simulink subsystem "Control_Attitude_Thrust"  (R2025b)
settings: Solver=VariableStepAuto  StartTime=0.0  StopTime=10.0  RelTol=1e-3
undefined symbols (not defined in the file): g0, Ktheta, Kthetadot, StabTrimPos, Tdoublet
libraries: simulink_extras x7
settings Model: Creator=invrt  LastModifiedBy=cdriggs

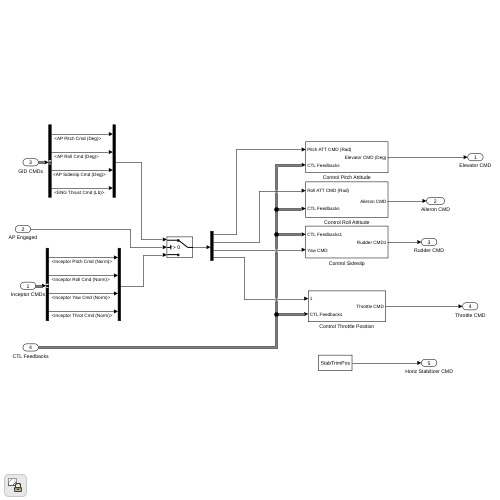
[thumbnail: Simulink's stored preview of the top-level diagram]
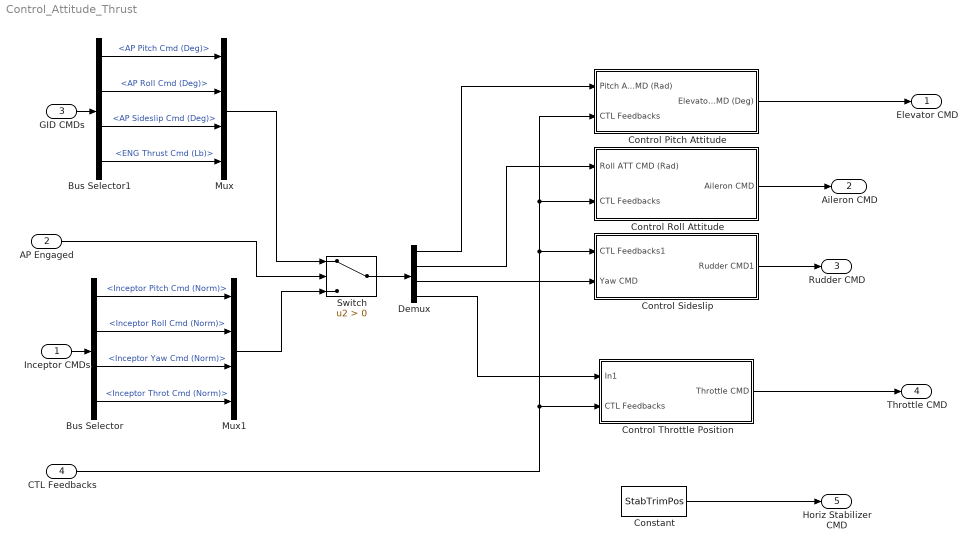
== system Control_Attitude_Thrust ==
  Inceptor CMDs : Inport
  AP Engaged : Inport  Port=2
  GID CMDs : Inport  Port=3
  CTL Feedbacks : Inport  Port=4
  Bus Selector : BusSelector  OutputSignals=Inceptor Pitch Cmd (Norm),Inceptor Roll Cmd (Norm),Inceptor Yaw Cmd (Norm),Inceptor Throt Cmd (Norm)
  Bus Selector1 : BusSelector  OutputSignals=AP Pitch Cmd (Deg),AP Roll Cmd (Deg),AP Sideslip Cmd (Deg),ENG Thrust Cmd (Lb)
  Constant : Constant  Value=StabTrimPos
  Control Pitch Attitude : Subsystem
  Control Roll Attitude : Subsystem
  Control Sideslip : Subsystem
  Control Throttle Position : Subsystem
  Demux : Demux
  Mux : Mux
  Mux1 : Mux
  Switch : Switch  Criteria=u2 > Threshold  SaturateOnIntegerOverflow=off  InputSameDT=off
  Elevator CMD : Outport
  Aileron CMD : Outport  Port=2
  Rudder CMD : Outport  Port=3
  Throttle CMD : Outport  Port=4
  Horiz Stabilizer CMD : Outport  Port=5
  wires:
  Inceptor CMDs/1 -> Bus Selector/1
  Bus Selector/1 -> Mux1/1  "<Inceptor Pitch Cmd (Norm)>"
  GID CMDs/1 -> Bus Selector1/1
  Bus Selector1/4 -> Mux/4  "<ENG Thrust Cmd (Lb)>"
  Bus Selector/2 -> Mux1/2  "<Inceptor Roll Cmd (Norm)>"
  Bus Selector1/2 -> Mux/2  "<AP Roll Cmd (Deg)>"
  Bus Selector1/1 -> Mux/1  "<AP Pitch Cmd (Deg)>"
  Bus Selector1/3 -> Mux/3  "<AP Sideslip Cmd (Deg)>"
  Bus Selector/3 -> Mux1/3  "<Inceptor Yaw Cmd (Norm)>"
  Bus Selector/4 -> Mux1/4  "<Inceptor Throt Cmd (Norm)>"
  AP Engaged/1 -> Switch/2
  Mux1/1 -> Switch/3
  Mux/1 -> Switch/1
  Demux/3 -> Control Sideslip/2(Yaw CMD)
  Demux/4 -> Control Throttle Position/1(In1)
  Control Throttle Position/1(Throttle CMD) -> Throttle CMD/1
  Control Sideslip/1(Rudder CMD1) -> Rudder CMD/1
  Constant/1 -> Horiz Stabilizer CMD/1
  CTL Feedbacks/1 -> Control Throttle Position/2(CTL Feedbacks), Control Pitch Attitude/2(CTL Feedbacks), Control Roll Attitude/2(CTL Feedbacks), Control Sideslip/1(CTL Feedbacks1)
  Demux/1 -> Control Pitch Attitude/1(Pitch ATT CMD (Rad))
  Demux/2 -> Control Roll Attitude/1(Roll ATT CMD (Rad))
  Control Pitch Attitude/1(Elevator CMD (Deg)) -> Elevator CMD/1
  Control Roll Attitude/1(Aileron CMD) -> Aileron CMD/1
  Switch/1 -> Demux/1

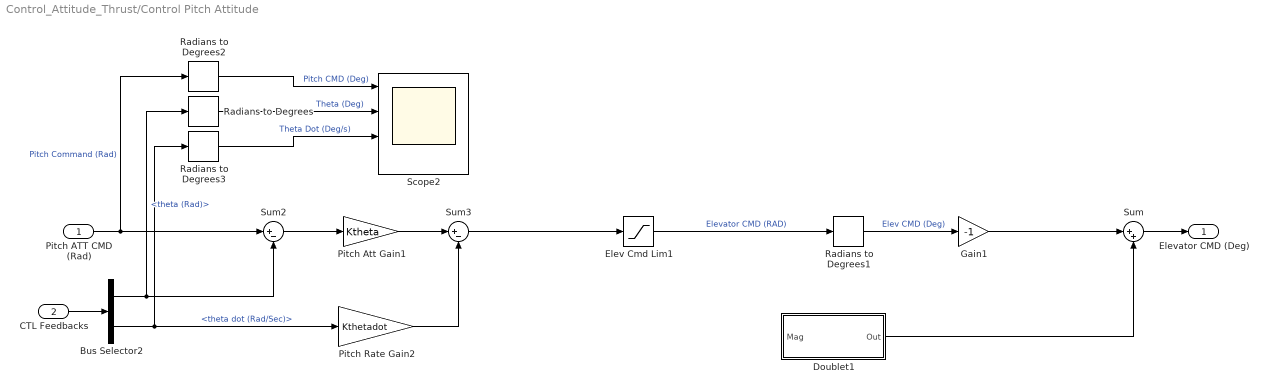
== system Control_Attitude_Thrust/Control Pitch Attitude ==
  Pitch ATT CMD (Rad) : Inport
  CTL Feedbacks : Inport  Port=2
  Bus Selector2 : BusSelector  OutputSignals=Rotat.Attitude.theta (Rad),Rotat.Attitude Rates.theta dot (Rad/Sec)
  Doublet1 : Subsystem
  Elev Cmd Lim1 : Saturate  UpperLimit=deg2rad(30)  LowerLimit=-deg2rad(30)
  Gain1 : Gain  Gain=-1
  Pitch Att Gain1 : Gain  Gain=Ktheta
  Pitch Rate Gain2 : Gain  Gain=Kthetadot
  Radians to Degrees{,1..3} (4 alike) : simulink_extras/Transformations/Radians to Degrees
  Scope2 : Scope  NumInputPorts=4
      settings: ActiveDisplayString=3  ActiveDisplayYMinimum=-21.350154604251  ActiveDisplayYMaximum=15.820828077072235  DataLoggingVariableName=ScopeData25
  Sum : Sum  Inputs=|++
  Sum2 : Sum  Inputs=|+-
  Sum3 : Sum  Inputs=|+-
  Elevator CMD (Deg) : Outport
  wires:
  Pitch Att Gain1/1 -> Sum3/1
  Pitch Rate Gain2/1 -> Sum3/2
  Radians to Degrees1/1 -> Gain1/1  "Elev CMD (Deg)"
  Sum3/1 -> Elev Cmd Lim1/1
  Sum2/1 -> Pitch Att Gain1/1
  Pitch ATT CMD (Rad)/1 -> Sum2/1, Radians to Degrees2/1  "Pitch Command (Rad)"
  Radians to Degrees/1 -> Scope2/2  "Theta (Deg)"
  Radians to Degrees2/1 -> Scope2/1  "Pitch CMD (Deg)"
  Elev Cmd Lim1/1 -> Radians to Degrees1/1  "Elevator CMD (RAD)"
  Radians to Degrees3/1 -> Scope2/3  "Theta Dot (Deg/s)"
  Doublet1/1(Out) -> Sum/2
  Sum/1 -> Elevator CMD (Deg)/1
  CTL Feedbacks/1 -> Bus Selector2/1
  Gain1/1 -> Sum/1
  Bus Selector2/1 -> Sum2/2, Radians to Degrees/1  "<theta (Rad)>"
  Bus Selector2/2 -> Pitch Rate Gain2/1, Radians to Degrees3/1  "<theta dot (Rad/Sec)>"

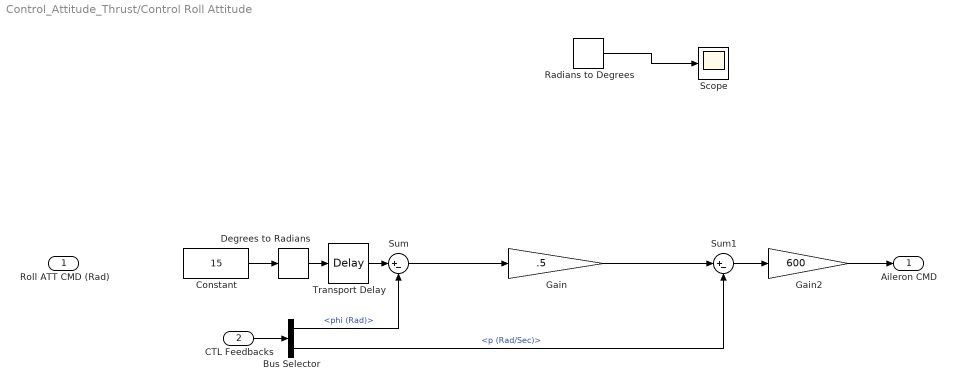
== system Control_Attitude_Thrust/Control Roll Attitude ==
  Roll ATT CMD (Rad) : Inport
  CTL Feedbacks : Inport  Port=2
  Bus Selector : BusSelector  OutputSignals=Rotat.Attitude.phi (Rad),Rotat.Body.Rates (Rad/Sec).p (Rad/Sec)
  Constant : Constant  Value=15
  Degrees to Radians : simulink_extras/Transformations/Degrees to Radians
  Gain : Gain  Gain=.5
  Gain2 : Gain  Gain=600
  Radians to Degrees : simulink_extras/Transformations/Radians to Degrees
  Scope : Scope
      settings: ActiveDisplayYMinimum=-1  ActiveDisplayYMaximum=1  DataLoggingVariableName=ScopeData2
  Sum : Sum  Inputs=|+-
  Sum1 : Sum  Inputs=|+-
  Transport Delay : TransportDelay  DelayTime=5
  Aileron CMD : Outport
  wires:
  Gain/1 -> Sum1/1
  Gain2/1 -> Aileron CMD/1
  Transport Delay/1 -> Sum/1
  Degrees to Radians/1 -> Transport Delay/1
  Sum1/1 -> Gain2/1
  Sum/1 -> Gain/1
  Constant/1 -> Degrees to Radians/1
  Radians to Degrees/1 -> Scope/1
  Bus Selector/1 -> Sum/2  "<phi (Rad)>"
  Bus Selector/2 -> Sum1/2  "<p (Rad/Sec)>"
  CTL Feedbacks/1 -> Bus Selector/1

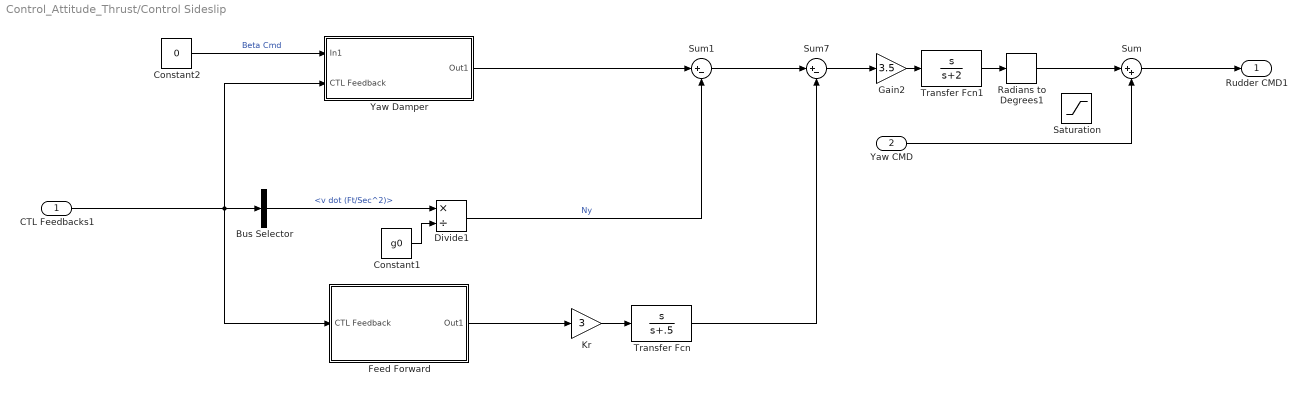
== system Control_Attitude_Thrust/Control Sideslip ==
  CTL Feedbacks1 : Inport
  Yaw CMD : Inport  Port=2
  Bus Selector : BusSelector  OutputSignals=Trans.Lin Accels.v dot (Ft/Sec^2)
  Constant1 : Constant  Value=g0
  Constant2 : Constant  Value=0
  Divide1 : Product  Inputs=*/
  Feed Forward : Subsystem
  Gain2 : Gain  Gain=3.5
  Kr : Gain  Gain=3
  Radians to Degrees1 : simulink_extras/Transformations/Radians to Degrees
  Saturation : Saturate  UpperLimit=3  LowerLimit=-3
  Sum : Sum  Inputs=|++
  Sum1 : Sum  Inputs=|+-
  Sum7 : Sum  Inputs=|+-
  Transfer Fcn : TransferFcn  Numerator=[1 0]  Denominator=[1 .5]
  Transfer Fcn1 : TransferFcn  Numerator=[1 0]  Denominator=[1 2]
  Yaw Damper : Subsystem
  Rudder CMD1 : Outport
  wires:
  Radians to Degrees1/1 -> Sum/1
  Sum/1 -> Rudder CMD1/1
  Transfer Fcn1/1 -> Radians to Degrees1/1
  Feed Forward/1(Out1) -> Kr/1
  Bus Selector/1 -> Divide1/1  "<v dot (Ft/Sec^2)>"
  Yaw CMD/1 -> Sum/2
  Gain2/1 -> Transfer Fcn1/1
  Yaw Damper/1(Out1) -> Sum1/1
  Sum1/1 -> Sum7/1
  Constant2/1 -> Yaw Damper/1(In1)  "Beta Cmd"
  Divide1/1 -> Sum1/2  "Ny"
  Kr/1 -> Transfer Fcn/1
  Constant1/1 -> Divide1/2
  CTL Feedbacks1/1 -> Bus Selector/1, Feed Forward/1(CTL Feedback), Yaw Damper/2(CTL Feedback)
  Sum7/1 -> Gain2/1
  Transfer Fcn/1 -> Sum7/2

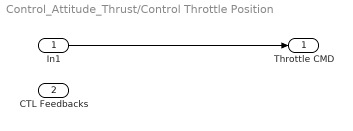
== system Control_Attitude_Thrust/Control Throttle Position ==
  In1 : Inport
  CTL Feedbacks : Inport  Port=2
  Throttle CMD : Outport
  wires:
  In1/1 -> Throttle CMD/1

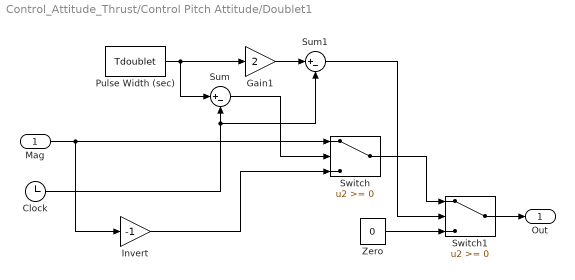
== system Control_Attitude_Thrust/Control Pitch Attitude/Doublet1 ==
  Mag : Inport
  Clock : Clock
  Gain1 : Gain  Gain=2
  Invert : Gain  Gain=-1
  Pulse Width (sec) : Constant  Value=Tdoublet
  Sum : Sum  Inputs=|+-
  Sum1 : Sum  Inputs=|+-
  Switch : Switch  SaturateOnIntegerOverflow=off  InputSameDT=off
  Switch1 : Switch  SaturateOnIntegerOverflow=off  InputSameDT=off
  Zero : Constant  Value=0
  Out : Outport
  wires:
  Sum1/1 -> Switch1/2
  Gain1/1 -> Sum1/1
  Switch1/1 -> Out/1
  Sum/1 -> Switch/2
  Clock/1 -> Sum/2, Sum1/2
  Zero/1 -> Switch1/3
  Switch/1 -> Switch1/1
  Invert/1 -> Switch/3
  Pulse Width (sec)/1 -> Gain1/1, Sum/1
  Mag/1 -> Invert/1, Switch/1

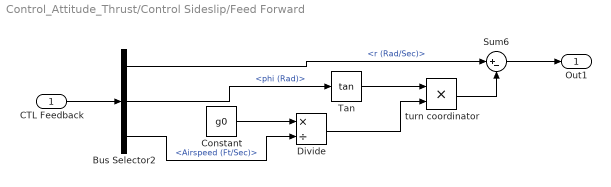
== system Control_Attitude_Thrust/Control Sideslip/Feed Forward ==
  CTL Feedback : Inport
  Bus Selector2 : BusSelector  OutputSignals=Rotat.Body.Rates (Rad/Sec).r (Rad/Sec),Rotat.Attitude.phi (Rad),Airspeed (Ft/Sec)
  Constant : Constant  Value=g0
  Divide : Product  Inputs=*/
  Sum6 : Sum  Inputs=|+-
  Tan : Trigonometry  Operator=tan
  turn coordinator : Product
  Out1 : Outport
  wires:
  CTL Feedback/1 -> Bus Selector2/1
  Bus Selector2/2 -> Tan/1  "<phi (Rad)>"
  Sum6/1 -> Out1/1
  turn coordinator/1 -> Sum6/2
  Divide/1 -> turn coordinator/2
  Bus Selector2/3 -> Divide/2  "<Airspeed (Ft/Sec)>"
  Constant/1 -> Divide/1
  Bus Selector2/1 -> Sum6/1  "<r (Rad/Sec)>"
  Tan/1 -> turn coordinator/1

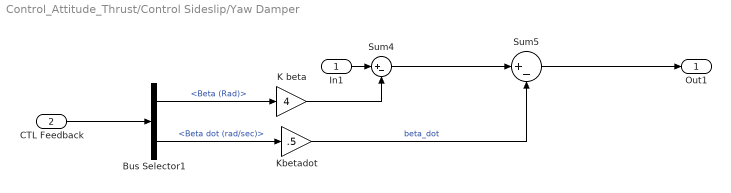
== system Control_Attitude_Thrust/Control Sideslip/Yaw Damper ==
  In1 : Inport
  CTL Feedback : Inport  Port=2
  Bus Selector1 : BusSelector  OutputSignals=Aero angles.Beta (Rad),Aero angles.Beta dot (rad/sec)
  K beta : Gain  Gain=4
  Kbetadot : Gain  Gain=.5
  Sum4 : Sum  Inputs=|+-
  Sum5 : Sum  Inputs=|+-
  Out1 : Outport
  wires:
  In1/1 -> Sum4/1
  CTL Feedback/1 -> Bus Selector1/1
  Kbetadot/1 -> Sum5/2  "beta_dot"
  Sum4/1 -> Sum5/1
  Bus Selector1/2 -> Kbetadot/1  "<Beta dot (rad/sec)>"
  Bus Selector1/1 -> K beta/1  "<Beta (Rad)>"
  Sum5/1 -> Out1/1
  K beta/1 -> Sum4/2
